simulink model "axis_servo"  (R2015a)
settings: Solver=ode45  StartTime=0.0  StopTime=10.0  RelTol=1e-3
undefined symbols (not defined in the file or in its folder): Ct, Dr, Jr, Mt
settings Model: Creator=shohei  LastModifiedBy=shohei

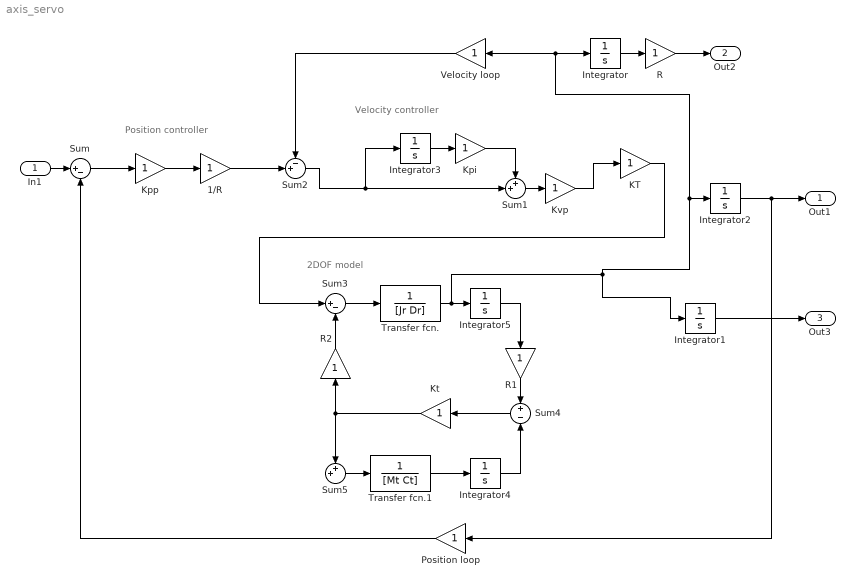
== system axis_servo ==
  note: 2DOF model
  note: Velocity controller
  note: Position controller
  In1 : Inport
  " Kt" : Gain
  1/R : Gain
  Integrator{,1..5} (6 alike) : Integrator
  KT : Gain
  Kpi : Gain
  Kpp : Gain
  Kvp : Gain
  Position loop : Gain
  R : Gain
  R1 : Gain
  R2 : Gain
  Sum : Sum  Inputs=|+-
  Sum1 : Sum  Inputs=++|
  Sum2 : Sum  Inputs=-+|
  Sum3 : Sum  Inputs=|+-
  Sum4 : Sum  Inputs=+|-
  Sum5 : Sum  Inputs=++|
  Transfer fcn. : TransferFcn  Denominator=[Jr Dr]
  Transfer fcn.1 : TransferFcn  Denominator=[Mt Ct]
  Velocity loop : Gain
  Out1 : Outport
  Out2 : Outport  Port=2
  Out3 : Outport  Port=3
  wires:
  In1/1 -> Sum/1
  Velocity loop/1 -> Sum2/1
  Integrator/1 -> R/1
  Transfer fcn./1 -> Integrator1/1, Integrator2/1, Velocity loop/1, Integrator/1, Integrator5/1
  R/1 -> Out2/1
  Integrator2/1 -> Position loop/1, Out1/1
  Integrator1/1 -> Out3/1
  Position loop/1 -> Sum/2
  1/R/1 -> Sum2/2
  Kvp/1 -> KT/1
  Sum/1 -> Kpp/1
  Kpp/1 -> 1/R/1
  Sum1/1 -> Kvp/1
  Sum2/1 -> Integrator3/1, Sum1/2
  Integrator3/1 -> Kpi/1
  Kpi/1 -> Sum1/1
  Integrator4/1 -> Sum4/2
  Transfer fcn.1/1 -> Integrator4/1
  KT/1 -> Sum3/1
  Sum5/1 -> Transfer fcn.1/1
  " Kt"/1 -> R2/1, Sum5/1
  Sum4/1 -> " Kt"/1
  Integrator5/1 -> R1/1
  R1/1 -> Sum4/1
  Sum3/1 -> Transfer fcn./1
  R2/1 -> Sum3/2
